simulink model "lab1_2"  (R2020b)
settings: Solver=VariableStepAuto  StartTime=0.0  StopTime=20  MaxStep=0.01  RelTol=1e-3
InitFcn:
  | lambda = 5;
  | theta = 5;
settings Model: Creator=Eeer12  LastModifiedBy=Eugene

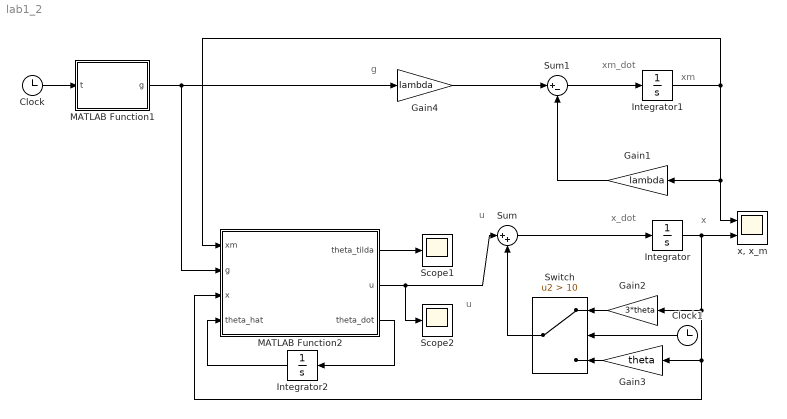
== system lab1_2 ==
  note: g
  note: u
  note: x_dot
  note: x
  note: xm_dot
  note: xm
  note: u
  Clock : Clock
  Clock1 : Clock
  Gain1 : Gain  Gain=lambda
  Gain2 : Gain  Gain=3*theta
  Gain3 : Gain  Gain=theta
  Gain4 : Gain  Gain=lambda
  Integrator : Integrator
  Integrator1 : Integrator
  Integrator2 : Integrator
  MATLAB Function1 : MATLAB Function  TreatAsAtomicUnit=on
  MATLAB Function2 : MATLAB Function  TreatAsAtomicUnit=on
  Scope1 : Scope
  Scope2 : Scope
  Sum : Sum  Inputs=|++
  Sum1 : Sum  Inputs=|+-
  Switch : Switch  Criteria=u2 > Threshold  Threshold=10
  "x, x_m" : Scope  NumInputPorts=2
  wires:
  Integrator/1 -> MATLAB Function2/3(x), Gain3/1, Gain2/1, "x, x_m"/2
  Sum/1 -> Integrator/1
  Gain1/1 -> Sum1/2
  Sum1/1 -> Integrator1/1
  Clock1/1 -> Switch/2
  Gain3/1 -> Switch/3
  Clock/1 -> MATLAB Function1/1(t)
  Integrator1/1 -> Gain1/1, "x, x_m"/1, MATLAB Function2/1(xm)
  Gain2/1 -> Switch/1
  Switch/1 -> Sum/2
  MATLAB Function2/2(u) -> Scope2/1, Sum/1
  MATLAB Function1/1(g) -> Gain4/1, MATLAB Function2/2(g)
  Gain4/1 -> Sum1/1
  MATLAB Function2/3(theta_dot) -> Integrator2/1
  Integrator2/1 -> MATLAB Function2/4(theta_hat)
  MATLAB Function2/1(theta_tilda) -> Scope1/1

== matlab function lab1_2/MATLAB Function1 ==
  data: t input; g output
function g = fcn(t)

g = 2*sin(5*t);

== matlab function lab1_2/MATLAB Function2 ==
  data: xm input; theta_tilda output; g input; x input; theta_hat input; u output; theta_dot output; lambda parameter; theta parameter
function [theta_tilda, u, theta_dot] = fcn(xm, g, x, theta_hat, lambda, theta)

gamma = 100;
e = xm - x;
theta_dot = -gamma*x*e;
u = -theta_hat*x - lambda*x + lambda*g;

theta_tilda = theta - theta_hat;
